simulink model "repressilator"  (R2018b)
settings: Solver=VariableStepAuto  StartTime=0.0  StopTime=100.0  RelTol=1e-3
libraries: Chip_Library x9
settings Model: Creator=phantom  LastModifiedBy=phantom

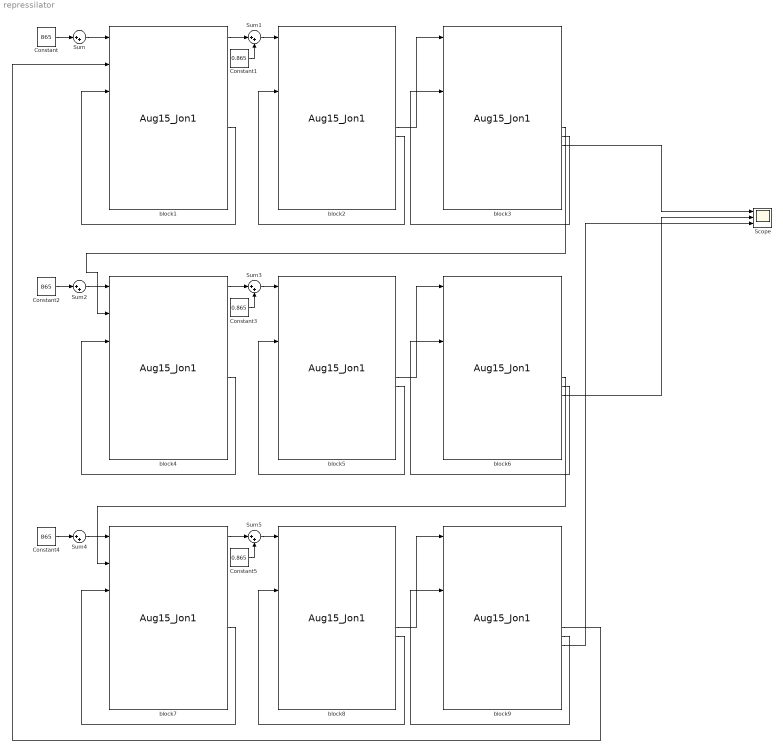
== system repressilator ==
  Constant : Constant  Value=865
  Constant1 : Constant  Value=0.865
  Constant2 : Constant  Value=865
  Constant3 : Constant  Value=0.865
  Constant4 : Constant  Value=865
  Constant5 : Constant  Value=0.865
  Scope : Scope  NumInputPorts=3
  Sum{,1..5} (6 alike) : Sum  Inputs=|++
  block1 : Chip_Library/Aug15_Jon1  Atot_cnst=0  Btot_cnst=0  Dfree_cnst=0  KDfw=4  KDrv=10  kr=1000  kdeg=1  ratC=0  n=2  c_ic=0.01  A_FB_EN=1  B_FB_EN=0  sel_rate=1  sel_Ctot=1
  block2 : Chip_Library/Aug15_Jon1  Atot_cnst=0  Btot_cnst=10  Dfree_cnst=10  KDfw=10  KDrv=10  kr=100  kdeg=1  ratC=0  n=1  c_ic=0.01  A_FB_EN=0  B_FB_EN=0  sel_rate=1  sel_Ctot=1
  block3 : Chip_Library/Aug15_Jon1  Atot_cnst=0  Btot_cnst=10  Dfree_cnst=10  KDfw=10  KDrv=10  kr=20  kdeg=1  ratC=0  n=1  c_ic=0.01  A_FB_EN=0  B_FB_EN=0  sel_rate=1  sel_Ctot=1
  block4 : Chip_Library/Aug15_Jon1  Atot_cnst=0  Btot_cnst=0  Dfree_cnst=0  KDfw=4  KDrv=10  kr=1000  kdeg=1  ratC=0  n=2  c_ic=0.01  A_FB_EN=1  B_FB_EN=0  sel_rate=1  sel_Ctot=1
  block5 : Chip_Library/Aug15_Jon1  Atot_cnst=0  Btot_cnst=10  Dfree_cnst=10  KDfw=10  KDrv=10  kr=100  kdeg=1  ratC=0  n=1  c_ic=0.01  A_FB_EN=0  B_FB_EN=0  sel_rate=1  sel_Ctot=1
  block6 : Chip_Library/Aug15_Jon1  Atot_cnst=0  Btot_cnst=10  Dfree_cnst=10  KDfw=10  KDrv=10  kr=20  kdeg=1  ratC=0  n=1  c_ic=0.01  A_FB_EN=0  B_FB_EN=0  sel_rate=1  sel_Ctot=1
  block7 : Chip_Library/Aug15_Jon1  Atot_cnst=0  Btot_cnst=0  Dfree_cnst=0  KDfw=4  KDrv=10  kr=1000  kdeg=1  ratC=0  n=2  c_ic=0.01  A_FB_EN=1  B_FB_EN=0  sel_rate=1  sel_Ctot=1
  block8 : Chip_Library/Aug15_Jon1  Atot_cnst=0  Btot_cnst=10  Dfree_cnst=10  KDfw=10  KDrv=10  kr=100  kdeg=1  ratC=0  n=1  c_ic=0.01  A_FB_EN=0  B_FB_EN=0  sel_rate=1  sel_Ctot=1
  block9 : Chip_Library/Aug15_Jon1  Atot_cnst=0  Btot_cnst=10  Dfree_cnst=10  KDfw=10  KDrv=10  kr=20  kdeg=1  ratC=0  n=1  c_ic=0.01  A_FB_EN=0  B_FB_EN=0  sel_rate=1  sel_Ctot=1
  wires:
  Constant/1 -> Sum/1
  Sum/1 -> block1/1
  Sum1/1 -> block2/1
  block1/1 -> Sum1/1
  Constant1/1 -> Sum1/2
  block1/11 -> block1/3
  block2/11 -> block3/1
  block2/12 -> block2/3
  block3/12 -> block3/3
  block6/12 -> block6/3
  block5/11 -> block6/1
  Constant3/1 -> Sum3/2
  Constant2/1 -> Sum2/1
  block4/1 -> Sum3/1
  block5/12 -> block5/3
  Sum3/1 -> block5/1
  Sum2/1 -> block4/1
  block4/11 -> block4/3
  block9/12 -> block9/3
  block8/11 -> block9/1
  Constant5/1 -> Sum5/2
  Constant4/1 -> Sum4/1
  block7/1 -> Sum5/1
  block8/12 -> block8/3
  Sum5/1 -> block8/1
  Sum4/1 -> block7/1
  block7/11 -> block7/3
  block3/11 -> block4/2
  block6/11 -> block7/2
  block3/13 -> Scope/1
  block6/13 -> Scope/2
  block9/11 -> block1/2
  block9/13 -> Scope/3
